simulink model "PID_Controller"  (R2020a)
settings: Solver=VariableStepAuto  StartTime=0.0  StopTime=10  RelTol=1e-3
settings Model: Creator=Prateek  LastModifiedBy=Prateek
settings DataIOCC: SaveOutput=off  SaveTime=off

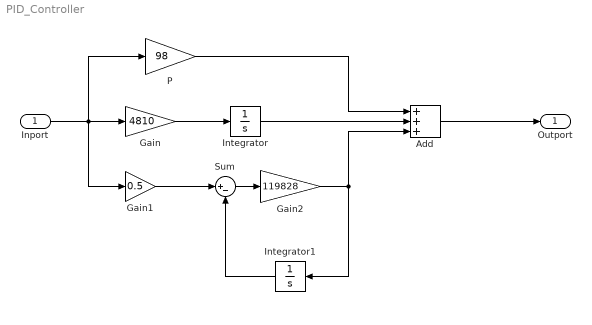
== system PID_Controller ==
  Inport : Inport  OutDataTypeStr=double  PortDimensions=1  SampleTime=0
  Add : Sum  Inputs=+++
  Gain : Gain  Gain=4810
  Gain1 : Gain  Gain=0.5
  Gain2 : Gain  Gain=119828
  Integrator : Integrator
  Integrator1 : Integrator
  P : Gain  Gain=98
  Sum : Sum  Inputs=|+-
  Outport : Outport  OutDataTypeStr=double  PortDimensions=1  SampleTime=0
  wires:
  Inport/1 -> Gain1/1, Gain/1, P/1
  Gain2/1 -> Integrator1/1, Add/3
  P/1 -> Add/1
  Integrator/1 -> Add/2
  Add/1 -> Outport/1
  Gain/1 -> Integrator/1
  Sum/1 -> Gain2/1
  Gain1/1 -> Sum/1
  Integrator1/1 -> Sum/2
